simulink subsystem "FL_FuselageForcesMoments"  (R2025a)
settings: Solver=VariableStepAuto  StartTime=0.0  StopTime=100  RelTol=1e-3
undefined symbols (not defined in the file): FL_AirDensity_P, FL_FuseLeverArm_P, FL_FuseXForces_M, FL_FuseXForces_X, FL_FuseXForces_Y, FL_FuseXMoment_M, FL_FuseXMoment_X, FL_FuseXMoment_Y, FL_FuseYForces_M, FL_FuseYForces_X, FL_FuseYForces_Y, FL_FuseYMoment_M, FL_FuseYMoment_X, FL_FuseYMoment_Y, FL_FuseZForces_M, FL_FuseZForces_X, FL_FuseZForces_Y, FL_FuseZMomentA_M, FL_FuseZMomentA_X, FL_FuseZMomentA_Y, FL_FuseZMomentB_M, FL_FuseZMomentB_X, FL_FuseZMomentB_Y, FL_PlanArea_P, FL_RotorRadius_P, FL_RotorWakeCoeff_P, FL_SideArea_P
settings Model: DataDictionary=Fuselage.sldd  EnableAccessToBaseWorkspace=off  DefaultTestHarness=FL_FuselagForcesMoments_Harness1  Creator=Admin  LastModifiedBy=Admin

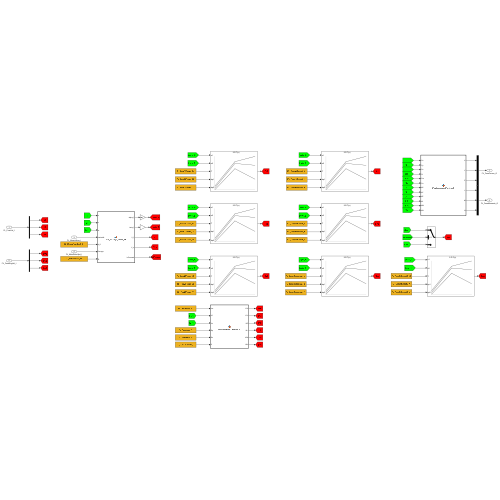
[thumbnail: Simulink's stored preview of the top-level diagram]
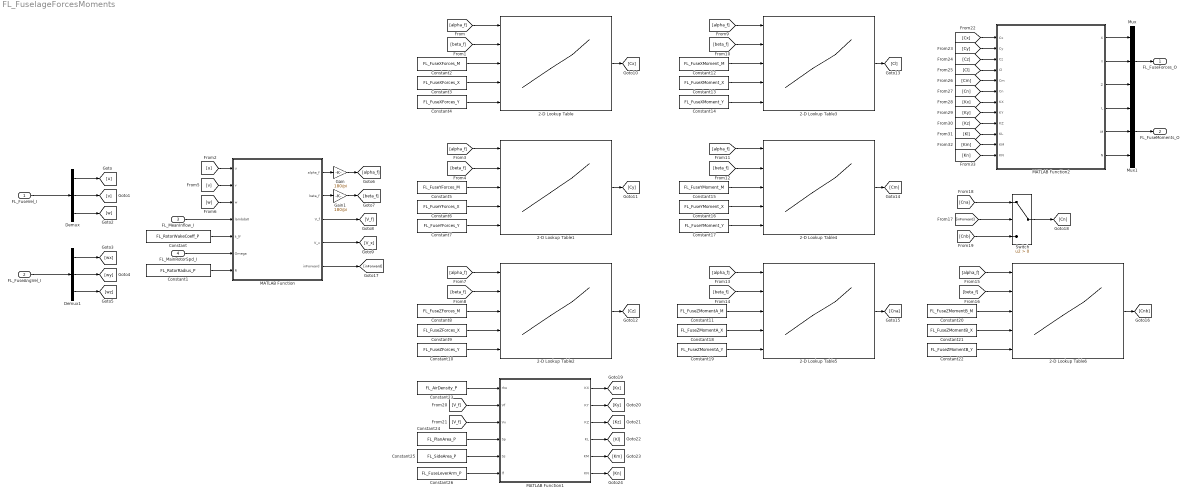
== system FL_FuselageForcesMoments ==
  FL_FuseVel_I : Inport
  FL_FuseAngVel_I : Inport  Port=2
  FL_MeanInflow_I : Inport  Port=3
  FL_MainRotorSpd_I : Inport  Port=4
  2-D Lookup Table{,1..6} (7 alike) : Lookup_n-D  BreakpointsForDimension1Source=Input port  BreakpointsForDimension1=[1:3]  BreakpointsForDimension2Source=Input port  BreakpointsForDimension2=[1:3]  TableSource=Input port  InternalRulePriority=Speed  RndMeth=Simplest
      settings: InputPortMap=u0,u1,p221,p5,p7
  Constant : Constant  Value=FL_RotorWakeCoeff_P
  Constant1 : Constant  Value=FL_RotorRadius_P
  Constant10 : Constant  Value=FL_FuseZForces_Y
  Constant11 : Constant  Value=FL_FuseZMomentA_M
  Constant12 : Constant  Value=FL_FuseXMoment_M
  Constant13 : Constant  Value=FL_FuseXMoment_X
  Constant14 : Constant  Value=FL_FuseXMoment_Y
  Constant15 : Constant  Value=FL_FuseYMoment_M
  Constant16 : Constant  Value=FL_FuseYMoment_X
  Constant17 : Constant  Value=FL_FuseYMoment_Y
  Constant18 : Constant  Value=FL_FuseZMomentA_X
  Constant19 : Constant  Value=FL_FuseZMomentA_Y
  Constant2 : Constant  Value=FL_FuseXForces_M
  Constant20 : Constant  Value=FL_FuseZMomentB_M
  Constant21 : Constant  Value=FL_FuseZMomentB_X
  Constant22 : Constant  Value=FL_FuseZMomentB_Y
  Constant23 : Constant  Value=FL_AirDensity_P
  Constant24 : Constant  Value=FL_PlanArea_P
  Constant25 : Constant  Value=FL_SideArea_P
  Constant26 : Constant  Value=FL_FuseLeverArm_P
  Constant3 : Constant  Value=FL_FuseXForces_X
  Constant4 : Constant  Value=FL_FuseXForces_Y
  Constant5 : Constant  Value=FL_FuseYForces_M
  Constant6 : Constant  Value=FL_FuseYForces_X
  Constant7 : Constant  Value=FL_FuseYForces_Y
  Constant8 : Constant  Value=FL_FuseZForces_M
  Constant9 : Constant  Value=FL_FuseZForces_X
  Demux : Demux  Outputs=3
  Demux1 : Demux  Outputs=3
  Gain : Gain  Gain=180/pi
  Gain1 : Gain  Gain=180/pi
  MATLAB Function : MATLAB Function  TreatAsAtomicUnit=on
  MATLAB Function1 : MATLAB Function  TreatAsAtomicUnit=on
  MATLAB Function2 : MATLAB Function  TreatAsAtomicUnit=on
  Mux : Mux  Inputs=3
  Mux1 : Mux  Inputs=3
  Switch : Switch  Criteria=u2 > Threshold  SaturateOnIntegerOverflow=off  InputSameDT=off
  FL_FuseForces_O : Outport
  FL_FuseMoments_O : Outport  Port=2
  wires:
  FL_FuseVel_I/1 -> Demux/1
  FL_FuseAngVel_I/1 -> Demux1/1
  Demux/1 -> [u]
  Demux/3 -> [w]
  Demux/2 -> [v]
  Demux1/1 -> [wx]
  Demux1/2 -> [wy]
  Demux1/3 -> [wz]
  FL_MeanInflow_I/1 -> MATLAB Function/4(lambda0)
  FL_MainRotorSpd_I/1 -> MATLAB Function/6(Omega)
  Constant/1 -> MATLAB Function/5(k_lf)
  Constant1/1 -> MATLAB Function/7(R)
  [u] -> MATLAB Function/1(u)
  [v] -> MATLAB Function/2(v)
  [w] -> MATLAB Function/3(w)
  MATLAB Function/1(alpha_f) -> Gain/1
  MATLAB Function/2(beta_f) -> Gain1/1
  MATLAB Function/4(V_x) -> [V_x]
  MATLAB Function/3(V_f) -> [V_f]
  [alpha_f] -> 2-D Lookup Table/1
  [beta_f] -> 2-D Lookup Table/2
  Constant2/1 -> 2-D Lookup Table/3
  Constant4/1 -> 2-D Lookup Table/5
  Constant3/1 -> 2-D Lookup Table/4
  2-D Lookup Table/1 -> [Cx]
  2-D Lookup Table1/1 -> [Cy]
  Constant6/1 -> 2-D Lookup Table1/4
  Constant7/1 -> 2-D Lookup Table1/5
  Constant5/1 -> 2-D Lookup Table1/3
  [beta_f] -> 2-D Lookup Table1/2
  [alpha_f] -> 2-D Lookup Table1/1
  [alpha_f] -> 2-D Lookup Table2/1
  [beta_f] -> 2-D Lookup Table2/2
  Constant8/1 -> 2-D Lookup Table2/3
  Constant10/1 -> 2-D Lookup Table2/5
  Constant9/1 -> 2-D Lookup Table2/4
  2-D Lookup Table2/1 -> [Cz]
  2-D Lookup Table5/1 -> [Cna]
  Constant18/1 -> 2-D Lookup Table5/4
  Constant19/1 -> 2-D Lookup Table5/5
  Constant11/1 -> 2-D Lookup Table5/3
  [beta_f] -> 2-D Lookup Table5/2
  [alpha_f] -> 2-D Lookup Table5/1
  [alpha_f] -> 2-D Lookup Table4/1
  [beta_f] -> 2-D Lookup Table4/2
  Constant15/1 -> 2-D Lookup Table4/3
  Constant17/1 -> 2-D Lookup Table4/5
  Constant16/1 -> 2-D Lookup Table4/4
  2-D Lookup Table4/1 -> [Cm]
  2-D Lookup Table3/1 -> [Cl]
  Constant13/1 -> 2-D Lookup Table3/4
  Constant14/1 -> 2-D Lookup Table3/5
  Constant12/1 -> 2-D Lookup Table3/3
  [beta_f] -> 2-D Lookup Table3/2
  [alpha_f] -> 2-D Lookup Table3/1
  [alpha_f] -> 2-D Lookup Table6/1
  [beta_f] -> 2-D Lookup Table6/2
  Constant20/1 -> 2-D Lookup Table6/3
  Constant22/1 -> 2-D Lookup Table6/5
  Constant21/1 -> 2-D Lookup Table6/4
  2-D Lookup Table6/1 -> [Cnb]
  MATLAB Function/5(inForward) -> [inForward]
  [inForward] -> Switch/2
  [Cna] -> Switch/1
  [Cnb] -> Switch/3
  Switch/1 -> [Cn]
  Constant23/1 -> MATLAB Function1/1(rho)
  [V_f] -> MATLAB Function1/2(Vf)
  Constant24/1 -> MATLAB Function1/4(Sp)
  Constant25/1 -> MATLAB Function1/5(Ss)
  Constant26/1 -> MATLAB Function1/6(lf)
  MATLAB Function1/1(KX) -> [Kx]
  MATLAB Function1/2(KY) -> [Ky]
  MATLAB Function1/3(KZ) -> [Kz]
  MATLAB Function1/4(KL) -> [Kl]
  MATLAB Function1/5(KM) -> [Km]
  MATLAB Function1/6(KN) -> [Kn]
  [V_f] -> MATLAB Function1/3(Vx)
  [Cx] -> MATLAB Function2/1(Cx)
  [Cy] -> MATLAB Function2/2(Cy)
  [Cz] -> MATLAB Function2/3(Cz)
  [Cl] -> MATLAB Function2/4(Cl)
  [Cm] -> MATLAB Function2/5(Cm)
  [Cn] -> MATLAB Function2/6(Cn)
  [Kx] -> MATLAB Function2/7(KX)
  [Ky] -> MATLAB Function2/8(KY)
  [Kz] -> MATLAB Function2/9(KZ)
  [Kl] -> MATLAB Function2/10(KL)
  [Km] -> MATLAB Function2/11(KM)
  [Kn] -> MATLAB Function2/12(KN)
  Mux/1 -> FL_FuseForces_O/1
  Mux1/1 -> FL_FuseMoments_O/1
  MATLAB Function2/2(Y) -> Mux/2
  MATLAB Function2/3(Z) -> Mux/3
  MATLAB Function2/1(X) -> Mux/1
  MATLAB Function2/4(L) -> Mux1/1
  MATLAB Function2/5(M) -> Mux1/2
  MATLAB Function2/6(N) -> Mux1/3
  Gain/1 -> [alpha_f]
  Gain1/1 -> [beta_f]

== matlab function FL_FuselageForcesMoments/MATLAB Function1 ==
  data: rho input; KX output; Vf input; Vx input; Sp input; Ss input; lf input; KY output; KZ output; KL output; KM output; KN output
function [KX, KY, KZ, KL, KM, KN] = FuselageAeroCoeffFactors(rho, Vf, Vx, Sp, Ss, lf)
%FUSELAGEAEROCOEFFFACORS Compute the multiplicative terms before
% aerodynamic coefficients for fuselage force and moment equations.
%
% Equations:
%   Xf = KX * Cxf(alpha_f, beta_f)
%   Yf = KY * Cyf(alpha_f, beta_f)
%   Zf = KZ * Czf(alpha_f, beta_f)
%   Lf = KL * Clf(alpha_f, beta_f)
%   Mf = KM * Cmf(alpha_f, beta_f)
%   Nf = KN * Cnf(alpha_f, beta_f)
%
% Inputs:
%   rho - air density [kg/m^3]
%   Vf  - effective fuselage airspeed [m/s]
%   Sp  - fuselage plan area [m^2]
%   Ss  - fuselage side area [m^2]
%   lf  - reference fuselage length [m]
%
% Outputs:
%   KX - factor before Cxf
%   KY - factor before Cyf
%   KZ - factor before Czf
%   KL - factor before Clf
%   KM - factor before Cmf
%   KN - factor before Cnf
%
% Notes:
%   Based on:
%       Xf = 1/2 * rho * Vf^2 * Sp     * Cxf
%       Yf = 1/2 * rho * Vf^2 * Ss     * Cyf
%       Zf = 1/2 * rho * Vf^2 * Sp     * Czf
%       Lf = 1/2 * rho * Vf^2 * Ss * lf * Clf
%       Mf = 1/2 * rho * Vf^2 * Sp * lf * Cmf
%       Nf = 1/2 * rho * Vf^2 * Ss * lf * Cnf

    qf = 0.5 .* rho .* Vf.^2;
    qx = 0.5 .* rho .* Vx.^2;

    KX = qx .* Sp;
    KY = qf .* Ss;
    KZ = qf .* Sp;

    KL = qf .* Ss .* lf;
    KM = qf .* Sp .* lf;
    KN = qf .* Ss .* lf;
end

== matlab function FL_FuselageForcesMoments/MATLAB Function ==
  data: u input; alpha_f output; beta_f output; v input; w input; lambda0 input; k_lf input; Omega input; R input; V_f output; V_x output; inForward output
function [alpha_f,beta_f, V_f, V_x, inForward] = calc_fuselage_alpha_Vf(u, v, w, lambda0, k_lf, Omega, R)
%CALC_FUSELAGE_ALPHA_VF Compute alpha_f and V_f from Padfield Eq. 3.241-3.243
%
% Inputs:
%   u, v, w - body-axis velocity components
%   lambda0 - mean inflow ratio
%   k_lf    - fuselage inflow interference factor
%   Omega   - rotor angular speed
%   R       - rotor radius
%
% Outputs:
%   alpha_f  - fuselage aerodynamic incidence angle [rad]
%   V_f      - effective fuselage speed
%   w_lambda - corrected vertical velocity term (NaN if lambda0 <= 0)
    inForward = u >= 0;
    if lambda0 > 0
        w_lambda = w - k_lf * Omega * R * lambda0;

    else
        w_lambda = w;

    end
    alpha_f = atan2(w_lambda, u);
    V_f = sqrt(u.^2 + v.^2 + w_lambda.^2);
    V_x = sqrt(u.^2 + w_lambda.^2);
    beta_f = asin(v/V_f);
end

== matlab function FL_FuselageForcesMoments/MATLAB Function2 ==
  data: Cx input; X output; Cy input; Cz input; Cl input; Cm input; Cn input; KX input; KY input; KZ input; KL input; KM input; KN input; Y output; Z output; L output; M output; N output
function [X, Y, Z, L, M, N] = FuselageLoadsFromCoeff( ...
    Cx, Cy, Cz, Cl, Cm, Cn, ...
    KX, KY, KZ, KL, KM, KN)
%FUSELAGELOADSFROMCOEFF Compute aerodynamic loads from coefficients and prefactors.
%
% Equations:
%   X = KX .* Cx
%   Y = KY .* Cy
%   Z = KZ .* Cz
%   L = KL .* Cl
%   M = KM .* Cm
%   N = KN .* Cn
%
% Inputs:
%   Cx, Cy, Cz - force coefficients
%   Cl, Cm, Cn - moment coefficients
%   KX, KY, KZ - force prefactors
%   KL, KM, KN - moment prefactors
%
% Outputs:
%   X, Y, Z - aerodynamic forces
%   L, M, N - aerodynamic moments
%
% Notes:
%   - Supports scalar, vector, or array inputs as long as sizes are compatible.
%   - Uses element-wise multiplication.

    X = KX .* Cx;
    Y = KY .* Cy;
    Z = KZ .* Cz;

    L = KL .* Cl;
    M = KM .* Cm;
    N = KN .* Cn;
end
